simulink model "线性系统simulink仿真"  (R2016b)
settings: Solver=FixedStepAuto  StartTime=0.0  StopTime=7  FixedStep=0.1  RelTol=1e-3
libraries: simulink x1
settings Model: Creator=Jake  LastModifiedBy=Jake

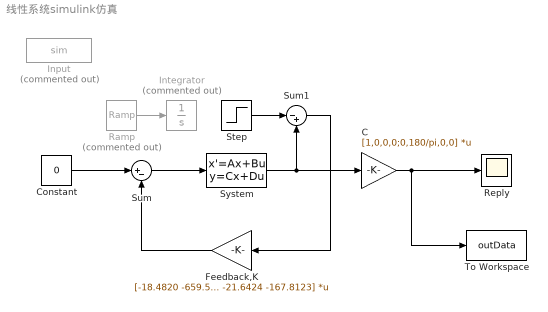
== system 线性系统simulink仿真 ==
  C : Gain  Gain=[1,0,0,0;0,180/pi,0,0]  Multiplication=Matrix(K*u)
  Constant : Constant  Value=0
  Feedback,K : Gain  Gain="[-18.4820 -659.5004  -21.6424 -167.8123]"  Multiplication=Matrix(K*u)
  Input : FromWorkspace  Commented=on  VariableName=sim  SampleTime=0
  Integrator : Integrator  Commented=on
  Ramp : simulink/Sources/Ramp  Commented=on  slope=0.1  start=0  X0=0
  Reply : Scope
  Step : Step  After=[10 5/180*pi 0 0]  SampleTime=0
  Sum : Sum  Inputs=|+-
  Sum1 : Sum  Inputs=|-+
  System : StateSpace  A=[0,0,1,0;0,0,0,1;0,-158.3,-0.07377,0;0,43.12,0.01615,0]  B=[0;0;0.9221;-0.2019]  C=[1,0,0,0;0,1,0,0;0,0,1,0;0,0,0,1]  D=[0;0;0;0]  X0=[0;0;0;0]
  To Workspace : ToWorkspace  VariableName=outData  SaveFormat=Structure With Time  SampleTime=-1
  wires:
  System/1 -> C/1, Sum1/2
  C/1 -> To Workspace/1, Reply/1
  Constant/1 -> Sum/1
  Sum/1 -> System/1
  Feedback,K/1 -> Sum/2
  Sum1/1 -> Feedback,K/1
  Ramp/1 -> Integrator/1
  Step/1 -> Sum1/1
